simulink model "b"  (R2018a)
settings: Solver=VariableStepAuto  StartTime=0.0  StopTime=10.0  RelTol=1e-3
libraries: commanabbnd3 x2
settings Model: Creator=Salman Prottoy  LastModifiedBy=Salman Prottoy

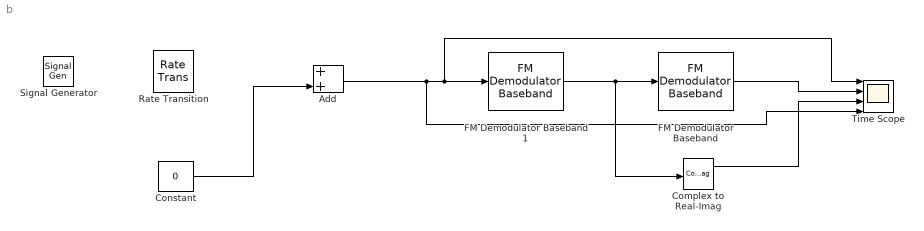
== system b ==
  "Add " : Sum
  "Complex to Real-Imag " : ComplexToRealImag
  "Constant " : Constant  Value=0
  "FM Demodulator Baseband " : commanabbnd3/FM Demodulator Baseband   FrequencyDeviation=100  SimulateUsing=Code generation
      settings: SourceProductName=Communications System Toolbox  SourceProductBaseCode=CM
  "FM Demodulator Baseband 1 " : commanabbnd3/FM Demodulator Baseband   FrequencyDeviation=75e3  SimulateUsing=Code generation
      settings: SourceProductName=Communications System Toolbox  SourceProductBaseCode=CM
  "Rate Transition " : RateTransition  OutPortSampleTime=1/100e3
  "Signal Generator " : SignalGenerator  Frequency=5
  Time Scope : Scope  NumInputPorts=4
  wires:
  "FM Demodulator Baseband "/1 -> Time Scope/2
  "Constant "/1 -> "Add "/2
  "FM Demodulator Baseband 1 "/1 -> "Complex to Real-Imag "/1, "FM Demodulator Baseband "/1
  "Add "/1 -> Time Scope/4, "FM Demodulator Baseband 1 "/1, Time Scope/1
  "Complex to Real-Imag "/1 -> Time Scope/3
